simulink subsystem "fin_forces_torques"  (R2025b)
settings: Solver=VariableStepAuto  StartTime=0.0  StopTime=10.0  RelTol=1e-3
undefined symbols (not defined in the file): fin_area, fin_aspectratio, fin_factor, fin_midchord_angle, fin_pos_x_cp, fin_pos_x_cp_mach2
settings Model: Creator=trist  LastModifiedBy=finnb

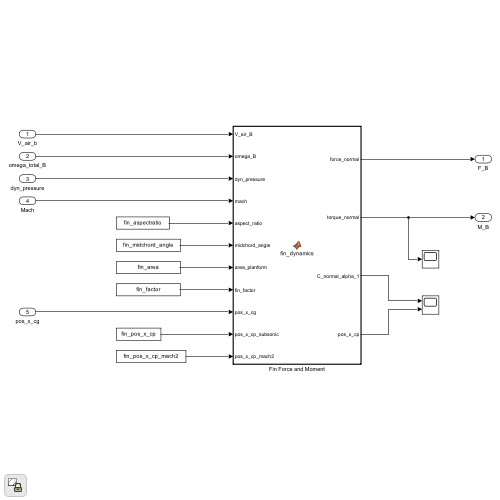
[thumbnail: Simulink's stored preview of the top-level diagram]
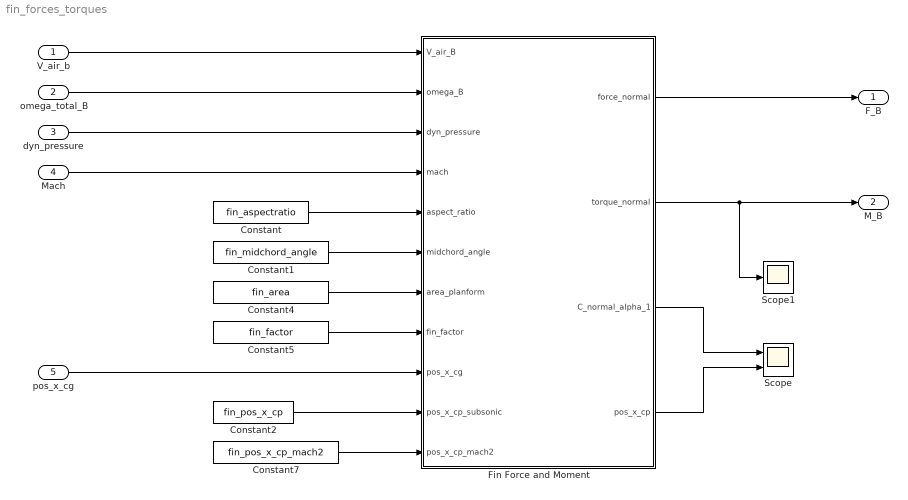
== system fin_forces_torques ==
  V_air_b : Inport
  omega_total_B : Inport  Port=2
  "dyn_pressure " : Inport  Port=3
  "Mach " : Inport  Port=4
  pos_x_cg : Inport  Port=5
  Constant : Constant  Value=fin_aspectratio
  Constant1 : Constant  Value=fin_midchord_angle
  Constant2 : Constant  Value=fin_pos_x_cp
  Constant4 : Constant  Value=fin_area
  Constant5 : Constant  Value=fin_factor
  Constant7 : Constant  Value=fin_pos_x_cp_mach2
  Fin Force and Moment : MATLAB Function  TreatAsAtomicUnit=on
  Scope : Scope  NumInputPorts=2
      settings: DataLoggingVariableName=ScopeData4
  Scope1 : Scope
      settings: DataLoggingVariableName=ScopeData13
  F_B : Outport
  M_B : Outport  Port=2  VectorParamsAs1DForOutWhenUnconnected=off
  wires:
  Constant/1 -> Fin Force and Moment/5(aspect_ratio)
  Constant1/1 -> Fin Force and Moment/6(midchord_angle)
  Constant4/1 -> Fin Force and Moment/7(area_planform)
  Constant5/1 -> Fin Force and Moment/8(fin_factor)
  Constant2/1 -> Fin Force and Moment/10(pos_x_cp_subsonic)
  pos_x_cg/1 -> Fin Force and Moment/9(pos_x_cg)
  Fin Force and Moment/3(C_normal_alpha_1) -> Scope/1
  Fin Force and Moment/1(force_normal) -> F_B/1
  "Mach "/1 -> Fin Force and Moment/4(mach)
  V_air_b/1 -> Fin Force and Moment/1(V_air_B)
  omega_total_B/1 -> Fin Force and Moment/2(omega_B)
  "dyn_pressure "/1 -> Fin Force and Moment/3(dyn_pressure)
  Fin Force and Moment/2(torque_normal) -> Scope1/1, M_B/1
  Fin Force and Moment/4(pos_x_cp) -> Scope/2
  Constant7/1 -> Fin Force and Moment/11(pos_x_cp_mach2)

== matlab function fin_forces_torques/Fin Force and Moment ==
  data: force_normal output; V_air_B input; omega_B input; dyn_pressure input; mach input; aspect_ratio input; midchord_angle input; area_planform input; fin_factor input; pos_x_cg input; torque_normal output; C_normal_alpha_1 output; pos_x_cp_subsonic input; pos_x_cp_mach2 input; pos_x_cp output
function [force_normal, torque_normal, C_normal_alpha_1, pos_x_cp] = fin_dynamics(V_air_B, omega_B, dyn_pressure, mach, aspect_ratio, midchord_angle, area_planform, fin_factor, pos_x_cg, pos_x_cp_subsonic, pos_x_cp_mach2)

    %%% Center of Pressure
    % threshold values
    subsonic = 0.6;
    supersonic = 1.6;

    % linear interpolation (for now)
    if mach <= subsonic
        pos_x_cp = pos_x_cp_subsonic;
    elseif mach >= supersonic 
        pos_x_cp = pos_x_cp_mach2;
    else % transonic
        pos_x_cp = (mach - supersonic) * (pos_x_cp_subsonic - pos_x_cp_mach2) / (subsonic - supersonic) + pos_x_cp_mach2;
    end

    pos_x = (pos_x_cp - pos_x_cg) * [1;0;0] + [0; 0.002; 0]; % + asymmetry


    %%% relative velocity
    Vrel = V_air_B + cross(omega_B, pos_x);

    % Body relative velocity magnitude
    Vrel_mag = norm(Vrel);
    Vrel_X = Vrel(1);
    Vrel_magYZ = norm(Vrel(2:3));
    incidence = atan2(Vrel_magYZ, Vrel_X);

    %%% calculate normal force coefficient
    C_normal_alpha_1 = aerosurface_online(mach, incidence, aspect_ratio, midchord_angle);

    %%% Forces
    if Vrel_magYZ ~= 0 % prevent division by 0
        % Angle of attack and component separation
        
        F_N_dir = [0; 
                   Vrel(2) / Vrel_magYZ; 
                   Vrel(3) / Vrel_magYZ];
        
        % Calculating total force
        F_N_mag = C_normal_alpha_1 * fin_factor * dyn_pressure * area_planform * sin(incidence);
        force_normal = F_N_dir * F_N_mag;
    else
        force_normal = [0; 0; 0];
    end

    % Total torque
    torque_normal = cross(force_normal, pos_x);

end
